simulink model "Model"  (R2026a)
settings: Solver=FixedStepDiscrete  StopTime=Tc*N_chirps  FixedStep=T_step
values from neighbouring files (symbols this model uses):
  c = 3e8    (= 300000000)    [radar_init.m]
  C_TVG = Max_Gain / (t_d_max^2)    (= 1e+18)    [radar_init.m]
  den_d = [1, (a-2)/(2+a)]    [radar_init.m]
  f0 = 0    [radar_init.m]
  fc = 77e9    (= 77000000000)    [radar_init.m]
  G_ADC_frontend = (Headroom_Fraction * V_FSR) / Measured_ADC_input_peak    [calibrate_adc_gain.m]    (also in radar_init.m = 1)
  K_target = sqrt(Prx_Ptx_ratio)    [radar_init.m]
  N_samples = Tc_steps / Clock_Divider    [radar_init.m]
  N_targets = length(R_target)    [radar_init.m]
  num_d = [a/(2+a), a/(2+a)]    [radar_init.m]
  R_target = [120]    [radar_init.m]
  S = B / Tc    (= 1.5e+13)    [radar_init.m]
  T_step = 1 / (10*B)    (= 6.66666666667e-10)    [radar_init.m]
  Tc = 10e-6    (= 1e-05)    [radar_init.m]
  Ts = Clock_Divider * T_step    [radar_init.m]
  v_target = [20]    [radar_init.m]
undefined symbols (not defined in the file or in its folder): dspblkCoreblockFVToolHelper, gcbh
libraries: dspxfrm3 x1, dspsigops x1
settings Model: Creator=daksh  LastModifiedBy=daksh

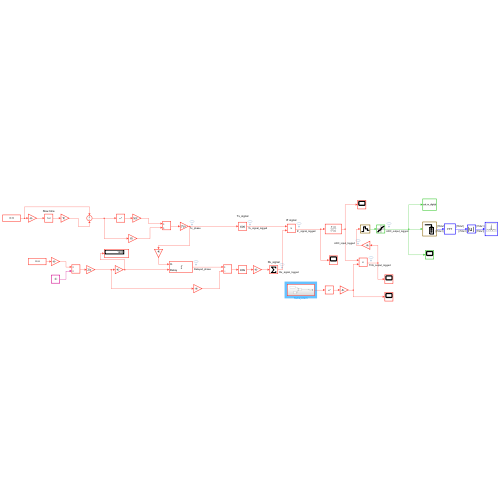
[thumbnail: Simulink's stored preview of the top-level diagram]
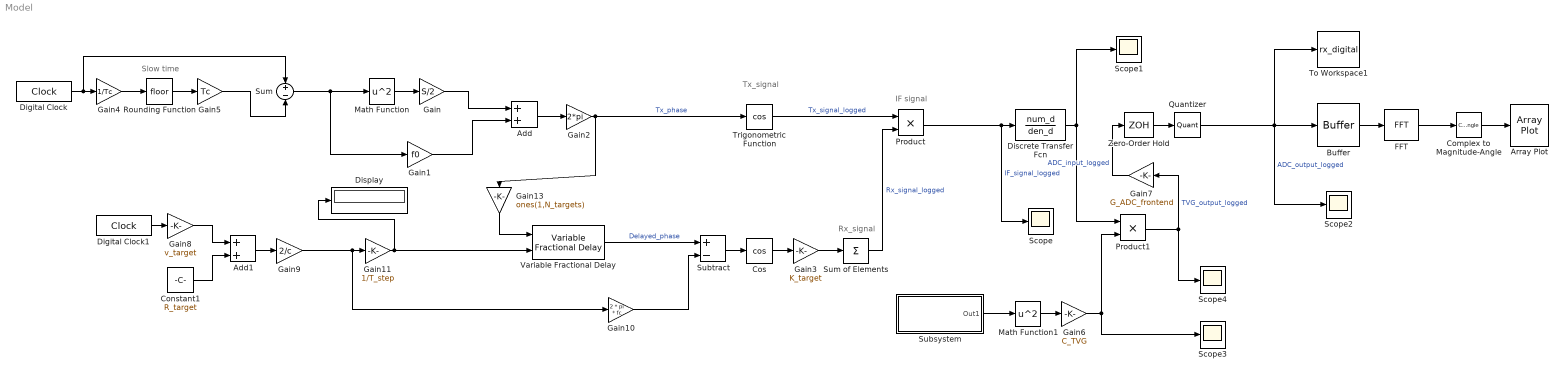
== system Model ==
  note: Slow time
  note: IF signal
  note: Rx_signal
  note: Tx_signal
  Add : Sum
  Add1 : Sum
  Array Plot : ArrayPlot  WindowPosition=[320.000000,200.000000,800.000000,500.000000,]  Visible=on  ScopeFrameLocation=window  MaximizeAxes=On  YLimits=[-209.5851 1904.1104]
  Buffer : Buffer  N=N_samples  OutputFrames=off
  Complex to Magnitude-Angle : ComplexToMagnitudeAngle  Output=Magnitude
  Constant1 : Constant  Value=R_target
  Cos : Trigonometry  Operator=cos
  Digital Clock : DigitalClock  SampleTime=T_step
  Digital Clock1 : DigitalClock  SampleTime=T_step
  Discrete Transfer Fcn : DiscreteTransferFcn  LoadFcn=dspblkCoreblockFVToolHelper(gcbh,'load');  Numerator=num_d  Denominator=den_d
      settings: CopyFcn=dspblkCoreblockFVToolHelper(gcbh,'copy');  DeleteFcn=dspblkCoreblockFVToolHelper(gcbh,'close');  ModelCloseFcn=dspblkCoreblockFVToolHelper(gcbh,'close');  PreSaveFcn=dspblkCoreblockFVToolHelper(gcbh,'presave');  PostSaveFcn=dspblkCoreblockFVToolHelper(gcbh,'postsave');  CloseFcn=dspblkCoreblockFVToolHelper(gcbh,'close');
  Display : Display
  FFT : dspxfrm3/FFT  FFTImplementation=Auto  CompMethod=Table lookup  TableOpt=NEW  TableOptActive=Speed  BitRevOrder=off  Normalize=off  InheritFFTLength=on  FFTLength=64  WrapInput=on  roundingMode=Ceiling  overflowMode=off  firstCoeffDataTypeStr=Inherit: Same word length as input  firstCoeffLastDataTypeStr=Inherit: Same word length as input  outputMin=[]  outputMax=[]
  Gain : Gain  Gain=S/2
  Gain1 : Gain  Gain=f0
  Gain10 : Gain  Gain=2 * pi * fc
  Gain11 : Gain  Gain=1/T_step
  Gain13 : Gain  Gain=ones(1,N_targets)
  Gain2 : Gain  Gain=2*pi
  Gain3 : Gain  Gain=K_target
  Gain4 : Gain  Gain=1/Tc
  Gain5 : Gain  Gain=Tc
  Gain6 : Gain  Gain=C_TVG
  Gain7 : Gain  Gain=G_ADC_frontend
  Gain8 : Gain  Gain=v_target
  Gain9 : Gain  Gain=2/c
  Math Function : Math  Operator=square
  Math Function1 : Math  Operator=square
  Product : Product
  Product1 : Product
  Quantizer : Quantizer  QuantizationInterval=Delta_q
  Rounding Function : Rounding
  Scope{,1..4} (5 alike) : Scope
      Scope settings: ActiveDisplayYMinimum=-1.9270786640344233E-6  ActiveDisplayYMaximum=1.8350252020775117E-6
      Scope1 settings: ActiveDisplayYMinimum=-1.8354146044948234E-6  ActiveDisplayYMaximum=1.8623661531941646E-6
      Scope2 settings: ActiveDisplayYMinimum=-1.3548014995478736E+7  ActiveDisplayYMaximum=1.4854806050604178E+7  DataLoggingVariableName=ScopeData2
      Scope3 settings: ActiveDisplayYMinimum=-2.6709209716121405E+6  ActiveDisplayYMaximum=1.01502188238093E+8  DataLoggingVariableName=ScopeData3
      Scope4 settings: ActiveDisplayYMinimum=-604.73598848363758  ActiveDisplayYMaximum=532.89062441105239  DataLoggingVariableName=ScopeData4
  Subsystem : Subsystem
  Subtract : Sum  Inputs=+-
  Sum : Sum  Inputs=+-
  Sum of Elements : Sum  Inputs=+
  To Workspace1 : ToWorkspace  VariableName=rx_digital  SampleTime=-1
      settings: Save2DSignal=2-D array (concatenate along first dimension)
  Trigonometric Function : Trigonometry  Operator=cos
  Variable Fractional Delay : dspsigops/Variable Fractional Delay  mode=OBSOLETE  modeActive=Linear  L=4  FarrowL=4  R=10  alpha=1  dmax=D_max_samples  InputProcessing=Columns as channels (frame based)  ic=0  noDFT=off  fallbackFIR=Clip to the minimum value necessary for centered kernel  fallbackFarrow=Clip to the minimum value necessary for centered kernel  roundingMode=Zero  overflowMode=off
  Zero-Order Hold : ZeroOrderHold  SampleTime=Ts
  wires:
  Math Function/1 -> Gain/1
  Gain/1 -> Add/1
  Add/1 -> Gain2/1
  Gain2/1 -> Trigonometric Function/1, Gain13/1  "Tx_phase"
  Gain3/1 -> Sum of Elements/1
  Zero-Order Hold/1 -> Quantizer/1
  Gain1/1 -> Add/2
  Quantizer/1 -> Scope2/1, Buffer/1, To Workspace1/1  "ADC_output_logged"
  Buffer/1 -> FFT/1
  FFT/1 -> Complex to Magnitude-Angle/1
  Complex to Magnitude-Angle/1 -> Array Plot/1
  Product/1 -> Discrete Transfer Fcn/1, Scope/1  "IF_signal_logged"
  Discrete Transfer Fcn/1 -> Product1/1, Scope1/1
  Digital Clock/1 -> Sum/1, Gain4/1
  Gain4/1 -> Rounding Function/1
  Rounding Function/1 -> Gain5/1
  Gain5/1 -> Sum/2
  Sum/1 -> Gain1/1, Math Function/1
  Math Function1/1 -> Gain6/1
  Product1/1 -> Gain7/1, Scope4/1  "TVG_output_logged"
  Gain6/1 -> Product1/2, Scope3/1
  Gain7/1 -> Zero-Order Hold/1  "ADC_input_logged"
  Constant1/1 -> Add1/2
  Gain8/1 -> Add1/1
  Add1/1 -> Gain9/1
  Gain9/1 -> Gain10/1, Gain11/1
  Subsystem/1(Out1) -> Math Function1/1
  Digital Clock1/1 -> Gain8/1
  Variable Fractional Delay/1 -> Subtract/1  "Delayed_phase"
  Subtract/1 -> Cos/1
  Gain10/1 -> Subtract/2
  Gain11/1 -> Variable Fractional Delay/2, Display/1
  Trigonometric Function/1 -> Product/1  "Tx_signal_logged"
  Cos/1 -> Gain3/1
  Gain13/1 -> Variable Fractional Delay/1
  Sum of Elements/1 -> Product/2  "Rx_signal_logged"

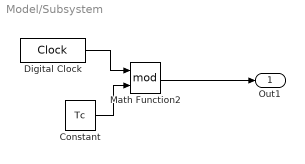
== system Model/Subsystem ==
  Constant : Constant  Value=Tc
  Digital Clock : DigitalClock  SampleTime=T_step
  Math Function2 : Math  Operator=mod
  Out1 : Outport
  wires:
  Math Function2/1 -> Out1/1
  Constant/1 -> Math Function2/2
  Digital Clock/1 -> Math Function2/1
